simulink model "ADIP_qLMPC"  (R2019a)
settings: Solver=ode4  StartTime=0.0  StopTime=param.Tsim  FixedStep=param.Ts  RelTol=1e-3
values from neighbouring files (symbols this model uses):
  switch_rA = 0    [run_qLMPC.m]
  Xko_init = kron(ones(param.N,1),zeros(4,1))    [run_qLMPC.m]
undefined symbols (not defined in the file or in its folder): param, sigbuilder_block
settings Model: Creator=pc  LastModifiedBy=ICS
settings DataIOCC: SaveFormat=StructureWithTime  ReturnWorkspaceOutputs=off
settings OptimizationCC: LifeSpan=inf
settings DebuggingCC: SFUnexpectedBacktrackingDiag=warning  SFNoUnconditionalDefaultTransitionDiag=warning  SFExecutionAtInitializationDiag=none  ArithmeticOperatorsInVariantConditions=warning
settings HardwareCC: ProdBitPerSizeT=32  ProdBitPerPtrDiffT=32  ProdWordSize=32  ProdHWDeviceType=Specified
settings SFSimCC: SimUseLocalCustomCode=off
settings RTWCC: RTWUseLocalCustomCode=off
settings CodeAppCC: StateflowObjectComments=on
settings GRTTargetCC: TargetLangStandard=C89/C90 (ANSI)  GeneratePreprocessorConditionals=Disable all
settings ConfigComp: CovMetricSettings=dw  CovHtmlReporting=on  CovSaveCumulativeToWorkspaceVar=on  CovSaveSingleToWorkspaceVar=on  CovExternalEMLEnable=off  CovSFcnEnable=off

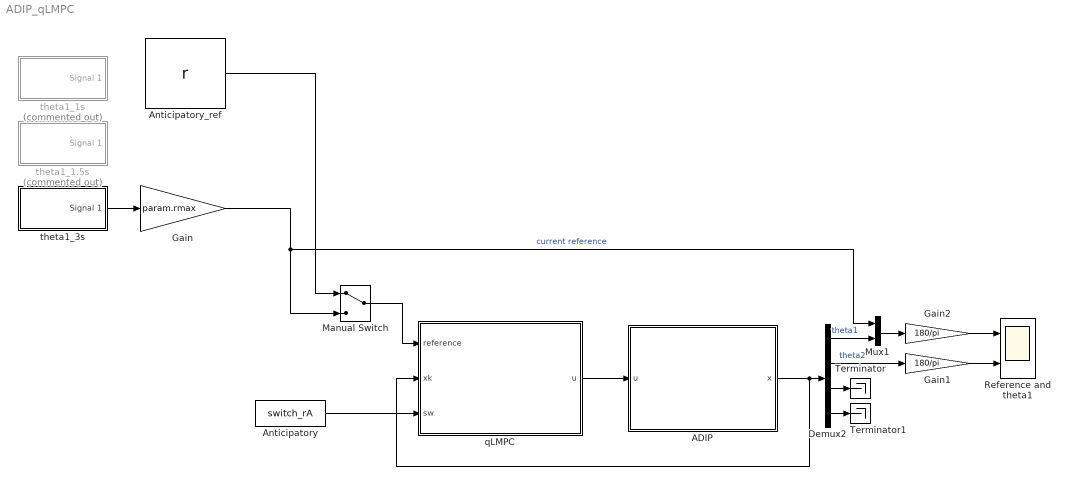
== system ADIP_qLMPC ==
  ADIP : Subsystem
  Anticipatory : Constant  Value=switch_rA
  Anticipatory_ref : FromWorkspace  VariableName=r  SampleTime=0
  Demux2 : Demux
  Gain : Gain  Gain=param.rmax
  Gain1 : Gain  Gain=180/pi
  Gain2 : Gain  Gain=180/pi
  Manual Switch : ManualSwitch
  Mux1 : Mux  Inputs=2
  Reference and theta1 : Scope  NumInputPorts=2
  Terminator : Terminator
  Terminator1 : Terminator
  qLMPC : Subsystem
  theta1_1.5s : Subsystem  Tag=STV Subsys  Commented=on  LoadFcn=sigbuilder_block('load');  StartFcn=sigbuilder_block('start');  StopFcn=sigbuilder_block('stop');  ClipboardFcn=sigbuilder_block('clipboard');  mask(Sigbuilder block){tuvar=[0:10]}
      mask help: Simulink:masks:SigbuilderBlock_MD
      mask init:
      | if ~strcmp(get_param(bdroot(gcbh),'SimulationStatus'),'stopped') tuvar = sigbuilder_block('maskInit'); end
      settings: CopyFcn=sigbuilder_block('copy');  DeleteFcn=sigbuilder_block('delete');  ModelCloseFcn=sigbuilder_block('modelClose');  PreSaveFcn=sigbuilder_block('preSave');  PauseFcn=sigbuilder_block('pause');  ContinueFcn=sigbuilder_block('continue');  NameChangeFcn=sigbuilder_block('namechange');  OpenFcn=sigbuilder_block('open',[5.5 30 1909 958 ]);  CloseFcn=sigbuilder_block('close');
      mask Display: plot(0, 0, 100, 100,[2, 2, 32, 32, 2], [68, 8, 8, 68, 68],[32, 2], [38, 38], [32, 19, 2],[53, 60, 44], [32, 17, 17, 2],[16, 16, 31, 31]);txt = getActiveGroup(gcbh);text(2, 100, txt,'verticalAlignment', 'top');
  theta1_1s : Subsystem  Tag=STV Subsys  Commented=on  LoadFcn=sigbuilder_block('load');  StartFcn=sigbuilder_block('start');  StopFcn=sigbuilder_block('stop');  ClipboardFcn=sigbuilder_block('clipboard');  mask(Sigbuilder block){tuvar=[0:10]}
      mask help: Simulink:masks:SigbuilderBlock_MD
      mask init:
      | if ~strcmp(get_param(bdroot(gcbh),'SimulationStatus'),'stopped') tuvar = sigbuilder_block('maskInit'); end
      settings: CopyFcn=sigbuilder_block('copy');  DeleteFcn=sigbuilder_block('delete');  ModelCloseFcn=sigbuilder_block('modelClose');  PreSaveFcn=sigbuilder_block('preSave');  PauseFcn=sigbuilder_block('pause');  ContinueFcn=sigbuilder_block('continue');  NameChangeFcn=sigbuilder_block('namechange');  OpenFcn=sigbuilder_block('open',[5.5 30 1909 958 ]);  CloseFcn=sigbuilder_block('close');
      mask Display: plot(0, 0, 100, 100,[2, 2, 32, 32, 2], [68, 8, 8, 68, 68],[32, 2], [38, 38], [32, 19, 2],[53, 60, 44], [32, 17, 17, 2],[16, 16, 31, 31]);txt = getActiveGroup(gcbh);text(2, 100, txt,'verticalAlignment', 'top');
  theta1_3s : Subsystem  Tag=STV Subsys  LoadFcn=sigbuilder_block('load');  StartFcn=sigbuilder_block('start');  StopFcn=sigbuilder_block('stop');  ClipboardFcn=sigbuilder_block('clipboard');  mask(Sigbuilder block){tuvar=[0:10]}
      mask help: Simulink:masks:SigbuilderBlock_MD
      mask init:
      | if ~strcmp(get_param(bdroot(gcbh),'SimulationStatus'),'stopped') tuvar = sigbuilder_block('maskInit'); end
      settings: CopyFcn=sigbuilder_block('copy');  DeleteFcn=sigbuilder_block('delete');  ModelCloseFcn=sigbuilder_block('modelClose');  PreSaveFcn=sigbuilder_block('preSave');  PauseFcn=sigbuilder_block('pause');  ContinueFcn=sigbuilder_block('continue');  NameChangeFcn=sigbuilder_block('namechange');  OpenFcn=sigbuilder_block('open',[5.5 30 1909 958 ]);  CloseFcn=sigbuilder_block('close');
      mask Display: plot(0, 0, 100, 100,[2, 2, 32, 32, 2], [68, 8, 8, 68, 68],[32, 2], [38, 38], [32, 19, 2],[53, 60, 44], [32, 17, 17, 2],[16, 16, 31, 31]);txt = getActiveGroup(gcbh);text(2, 100, txt,'verticalAlignment', 'top');
  wires:
  Demux2/1 -> Mux1/2  "theta1"
  Demux2/2 -> Gain1/1  "theta2"
  Mux1/1 -> Gain2/1
  theta1_3s/1(Signal 1) -> Gain/1
  Gain1/1 -> Reference and theta1/2
  Gain2/1 -> Reference and theta1/1
  ADIP/1(x) -> qLMPC/2(xk), Demux2/1
  qLMPC/1(u) -> ADIP/1(u)
  Demux2/4 -> Terminator1/1
  Demux2/3 -> Terminator/1
  Gain/1 -> Mux1/1, Manual Switch/2  "current reference"
  Anticipatory/1 -> qLMPC/3(sw)
  Manual Switch/1 -> qLMPC/1(reference)
  Anticipatory_ref/1 -> Manual Switch/1

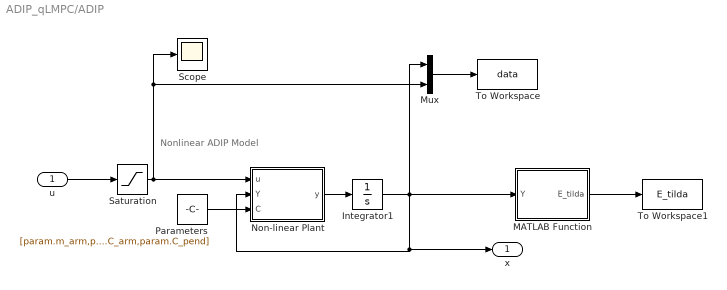
== system ADIP_qLMPC/ADIP ==
  note: Nonlinear ADIP Model
  u : Inport
  Integrator1 : Integrator  InitialCondition=param.theta0
  MATLAB Function : MATLAB Function  TreatAsAtomicUnit=on
  Mux : Mux  Inputs=2
  "Non-linear Plant " : MATLAB Function  TreatAsAtomicUnit=on
  Parameters : Constant  Value=[param.m_arm,param.m_pend,param.m_hinge,param.l_pivot,param.l_pend,param.g,param.Jarm,param.Jpend,param.Jl,param.Jhinge, param.C_arm,param.C_pend]
  Saturation : Saturate  UpperLimit=2.5  LowerLimit=-2.5
  Scope : Scope
  To Workspace : ToWorkspace  VariableName=data  SampleTime=-1
  To Workspace1 : ToWorkspace  VariableName=E_tilda  SampleTime=-1
  x : Outport
  wires:
  "Non-linear Plant "/1(y) -> Integrator1/1
  Parameters/1 -> "Non-linear Plant "/3(C)
  Mux/1 -> To Workspace/1
  Saturation/1 -> Mux/2, Scope/1, "Non-linear Plant "/1(u)
  u/1 -> Saturation/1
  Integrator1/1 -> Mux/1, "Non-linear Plant "/2(Y), x/1, MATLAB Function/1(Y)
  MATLAB Function/1(E_tilda) -> To Workspace1/1

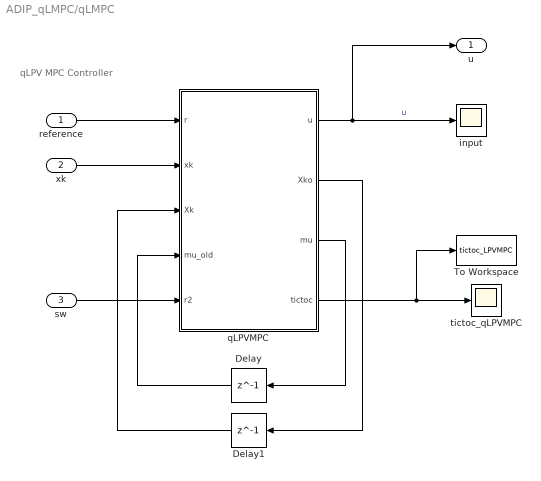
== system ADIP_qLMPC/qLMPC ==
  note: qLPV MPC Controller
  reference : Inport
  xk : Inport  Port=2
  sw : Inport  Port=3
  Delay : Delay  DelayLength=1  InitialCondition=zeros(2*param.N,1)
  Delay1 : Delay  DelayLength=1  InitialCondition=Xko_init
  To Workspace : ToWorkspace  VariableName=tictoc_LPVMPC  SaveFormat=Timeseries  SampleTime=-1
  input : Scope
  qLPVMPC : MATLAB Function  TreatAsAtomicUnit=on
  tictoc_qLPVMPC : Scope
  u : Outport
  wires:
  qLPVMPC/1(u) -> u/1, input/1  "u"
  Delay/1 -> qLPVMPC/4(mu_old)
  qLPVMPC/3(mu) -> Delay/1
  Delay1/1 -> qLPVMPC/3(Xk)
  qLPVMPC/2(Xko) -> Delay1/1
  qLPVMPC/4(tictoc) -> To Workspace/1, tictoc_qLPVMPC/1
  xk/1 -> qLPVMPC/2(xk)
  reference/1 -> qLPVMPC/1(r)
  sw/1 -> qLPVMPC/5(r2)

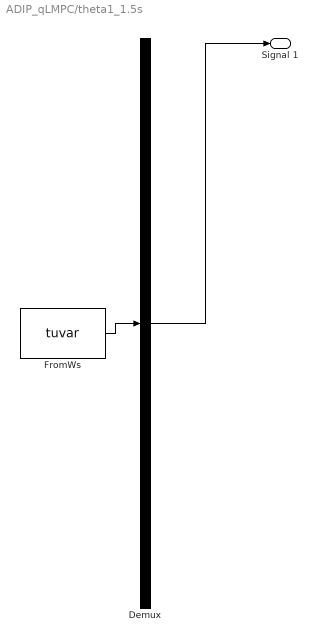
== system ADIP_qLMPC/theta1_1.5s ==
  Demux : Demux  Tag=STV Demux  Outputs=1
  FromWs : FromWorkspace  Tag=STV FromWs  VariableName=tuvar  SampleTime=0
      SigBuilderData=|
      | common.afterFinalStr = 'Extrapolate'
      | common.sampleTime = 0
      | dataSet.timeRange = [0 50]
      | dataSet.name = 'Group 1'
      | sbobj.Groups.Name = 'Group 1'
      | sbobj.Groups.Signals.Name = 'Signal 1'
      | sbobj.Groups.Signals.XData = [0 2 3.5 6.5 9.5 12.5 14 50]
      | sbobj.Groups.Signals.YData = [0 0 1 1 -1 -1 0 0]
      | sbobj.Groups.TimeRange = [0 50]
  Signal 1 : Outport  Tag=STV Outport
  wires:
  Demux/1 -> Signal 1/1
  FromWs/1 -> Demux/1

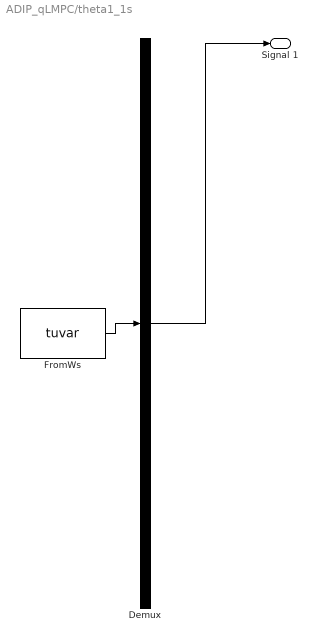
== system ADIP_qLMPC/theta1_1s ==
  Demux : Demux  Tag=STV Demux  Outputs=1
  FromWs : FromWorkspace  Tag=STV FromWs  VariableName=tuvar  SampleTime=0
      SigBuilderData=|
      | common.afterFinalStr = 'Extrapolate'
      | common.sampleTime = 0
      | dataSet.timeRange = [0 50]
      | dataSet.name = 'Group 1'
      | sbobj.Groups.Name = 'Group 1'
      | sbobj.Groups.Signals.Name = 'Signal 1'
      | sbobj.Groups.Signals.XData = [0 2 3 6.5 8.5 12.5 13.5 50]
      | sbobj.Groups.Signals.YData = [0 0 1 1 -1 -1 0 0]
      | sbobj.Groups.TimeRange = [0 50]
  Signal 1 : Outport  Tag=STV Outport
  wires:
  Demux/1 -> Signal 1/1
  FromWs/1 -> Demux/1

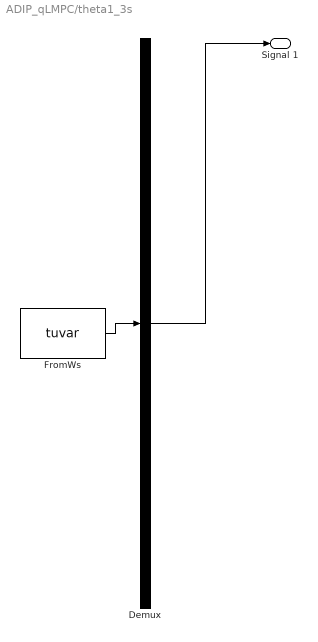
== system ADIP_qLMPC/theta1_3s ==
  Demux : Demux  Tag=STV Demux  Outputs=1
  FromWs : FromWorkspace  Tag=STV FromWs  VariableName=tuvar  SampleTime=0
      SigBuilderData=|
      | common.afterFinalStr = 'Extrapolate'
      | common.sampleTime = 0
      | dataSet.timeRange = [0 50]
      | dataSet.name = 'Group 1'
      | sbobj.Groups.Name = 'Group 1'
      | sbobj.Groups.Signals.Name = 'Signal 1'
      | sbobj.Groups.Signals.XData = [0 2 5 6.5 10.5 12 15 50]
      | sbobj.Groups.Signals.YData = [0 0 1 1 -1 -1 0 0]
      | sbobj.Groups.TimeRange = [0 50]
  Signal 1 : Outport  Tag=STV Outport
  wires:
  Demux/1 -> Signal 1/1
  FromWs/1 -> Demux/1

== matlab function ADIP_qLMPC/ADIP/Non-linear Plant  ==
  data: u input; Y input; y output; C input
function y = fcn(u,Y,C)
m1=C(1); % Mass of arm
m2=C(2); % Mass of pendulum
mh = C(3); % Mass of Hinge
l1  = C(4); % Length of arm
l2 = C(5); % Length of pendulum
g_ = C(6);
J_arm = C(7);
J_pend = C(8);
J_motor = C(9);
J_sensor = C(10);
fv1 = C(11);
fv2 = C(12);

y1 = Y(1);  % actual theta1          
y2 = Y(2);  % actual theta2
y3 = Y(3);  % actual theta1d
y4 = Y(4);  % actual theta2d

dy1 = y3;
dy2 = y4;
dy3 =-(2*(8*J_pend*fv1*y3 - 2*l2^2*m2*u - 8*J_pend*u + 2*fv1*l2^2*m2*y3 + l1^2*l2^2*m2^2*y3^2*sin(2*y1 - 2*y2) + l1*l2^3*m2^2*y4^2*sin(y1 - y2) + g_*l1*l2^2*m2^2*sin(y1) + 4*J_pend*g_*l1*m1*sin(y1) + 8*J_pend*g_*l1*m2*sin(y1) + 8*J_pend*g_*l1*mh*sin(y1) + g_*l1*l2^2*m2^2*sin(y1 - 2*y2) - 4*fv2*l1*l2*m2*y4*cos(y1 - y2) + g_*l1*l2^2*m1*m2*sin(y1) + 2*g_*l1*l2^2*m2*mh*sin(y1) + 4*J_pend*l1*l2*m2*y4^2*sin(y1 - y2)))/(16*J_arm*J_pend + 16*J_motor*J_pend + 16*J_pend*J_sensor + 4*l1^2*l2^2*m2^2 + 4*J_arm*l2^2*m2 + 4*J_motor*l2^2*m2 + 4*J_pend*l1^2*m1 + 16*J_pend*l1^2*m2 + 4*J_sensor*l2^2*m2 - 4*l1^2*l2^2*m2^2*cos(y1 - y2)^2 + l1^2*l2^2*m1*m2);
dy4 =(2*(l1^2*l2^2*m2^2*y4^2*sin(2*y1 - 2*y2) - 8*J_motor*fv2*y4 - 8*J_sensor*fv2*y4 - 2*fv2*l1^2*m1*y4 - 8*fv2*l1^2*m2*y4 - 8*J_arm*fv2*y4 - 4*l1*l2*m2*u*cos(y1 - y2) + 2*g_*l1^2*l2*m2^2*sin(2*y1 - y2) + 4*l1^3*l2*m2^2*y3^2*sin(y1 - y2) - 2*g_*l1^2*l2*m2^2*sin(y2) - 4*J_arm*g_*l2*m2*sin(y2) - 4*J_motor*g_*l2*m2*sin(y2) - 4*J_sensor*g_*l2*m2*sin(y2) + g_*l1^2*l2*m1*m2*sin(2*y1 - y2) + 2*g_*l1^2*l2*m2*mh*sin(2*y1 - y2) + l1^3*l2*m1*m2*y3^2*sin(y1 - y2) + 4*fv1*l1*l2*m2*y3*cos(y1 - y2) + 2*g_*l1^2*l2*m2*mh*sin(y2) + 4*J_arm*l1*l2*m2*y3^2*sin(y1 - y2) + 4*J_motor*l1*l2*m2*y3^2*sin(y1 - y2) + 4*J_sensor*l1*l2*m2*y3^2*sin(y1 - y2)))/(16*J_arm*J_pend + 16*J_motor*J_pend + 16*J_pend*J_sensor + 2*l1^2*l2^2*m2^2 + 4*J_arm*l2^2*m2 + 4*J_motor*l2^2*m2 + 4*J_pend*l1^2*m1 + 16*J_pend*l1^2*m2 + 4*J_sensor*l2^2*m2 - 2*l1^2*l2^2*m2^2*cos(2*y1 - 2*y2) + l1^2*l2^2*m1*m2);
y = [dy1 dy2 dy3 dy4]';

== matlab function ADIP_qLMPC/qLMPC/qLPVMPC ==
  settings: updateMethod=DISCRETE  sampleTime=0.01
  data: r input; xk input size=4; u output; Xko output; mu output; tictoc output; Xk input; mu_old input; r2 input; param parameter
function [u,Xko,mu,tictoc]= qLPVMPC(r,xk,Xk,mu_old,r2,param)
% Code adapted to requirements from the original file by Pablo S.G.
% Cisneros and Antje Dittmer. Neither integral action nor a disturbance
% model is considered in this code.

% MATLAB_Function calculates controller output u. It turns the QP into a 
% linear complementarity problem (LCP) and solves it with Lemke's algorithm.
%
% Inputs: * r: reference
%         * xk: quasiLPV KF state estimates
%         * Xk: Xko(= L*xk+S*U) delayed by one sample timestep
%         * mu_old: mu delayed by one sample timestep
%         * sysConst: system constants of pendulum (lengths, masses, etc.)
%         
% Outputs: * u: controller output at current time step
%          * Xko: Future state trajectory (L*xk+S*U)
%          * mu: Result Lemke's algorithm/LCP: M mu +q >=0, mu>=0, mu'(Mmu+q)=0
%          * us: xuss(end) from xuss = [eye(4)-Ass -Bss;[1 0 0 0] 0]\[Bss*d;1]
%          * tictoc: tic-toc result

% Pablo S.G. Cisneros, Herbert Werner, ICS TUHH

%#codegen
coder.extrinsic('tic');
coder.extrinsic('toc');
tictoc = 0;
tic
%% Init N, Q, R
N = 40; % CHANGE THIS PARAMETER CORRESPONDING TO THE MAIN FILE
q_ = param.Q;
R_ = param.R*eye(N); 
p = param.P; 
U = zeros(N,1);
nx = length(xk);
Ulim = param.Ulim * ones(2*N,1);
Ts = param.Ts;
iterations = 1;
if r2 % Anticipatory reference signal
    ref = r;
else % current reference signal
    ref = repmat([r; 0; 0; 0],N,1); %ref = kron(ones(N,1),[r; 0; 0; 0;0]); 
end
%% Shift Xk
Xk(1:end-nx) = Xk(nx+1:end); 
for i = 1:iterations
    [L,S,H,g] = HSqLd(N,q_,R_,p,xk,Xk,Ts,ref,param);

    %% %%%%%%Turn QP into LCP and solve it%%%%%%%%%
    Ac_ = [-eye(N);eye(N)];
    bc_ = - Ulim;
    Hi = eye(size(H,1))/H;
    M = Ac_*Hi*Ac_';
    q = -Ac_*Hi*g - bc_;
 
    mu = lemke(M,q,mu_old);
 
    U = Hi*(Ac_'*mu-g);
    U(isnan(U)) = 0;
    
    %% %%%%%%%%%%%%%%%%%%%%%%%%%%%%%%%%%%%%%%%%%%%%    
    Xko = L*xk+S*U;
end
u =  U(1);

tictoc = toc;

== matlab function ADIP_qLMPC/ADIP/MATLAB Function ==
  data: Y input; E_tilda output; param parameter
function E_tilda = fcn(Y,param)

m1 = param.m_arm;
m2 = param.m_pend;
mh = param.m_hinge;
l1 = param.l_pivot;
l2 = param.l_pend;
g_ = param.g;
J_arm = param.Jarm;
J_pend = param.Jpend;
J_motor = param.Jl;
J_sensor = param.Jhinge;

y1 = Y(1);  % actual theta1          
y2 = Y(2);  % actual theta2
y3 = Y(3);  % actual theta1d
y4 = Y(4);  % actual theta2d
E_tilda = (J_arm*y3^2)/2 + (J_motor*y3^2)/2 + (J_pend*y4^2)/2 + (J_sensor*y3^2)/2 + g_*m1*(l1/2 - (l1*cos(y1))/2) + g_*m2*(l1 + l2/2 - l1*cos(y1) - (l2*cos(y2))/2) + g_*mh*(l1 - l1*cos(y1));
